simulink library "csu_tmp_tracker_messsage_processing_lib"  (R2014b)
settings: Solver=ode45  StartTime=0.0  StopTime=10.0  RelTol=1e-3
libraries: util_info_lib x1
settings Model: Creator=escrane  LastModifiedBy=mstewart

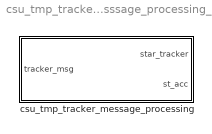
== system csu_tmp_tracker_messsage_processing_lib ==
  csu_tmp_tracker_message_processing : Subsystem

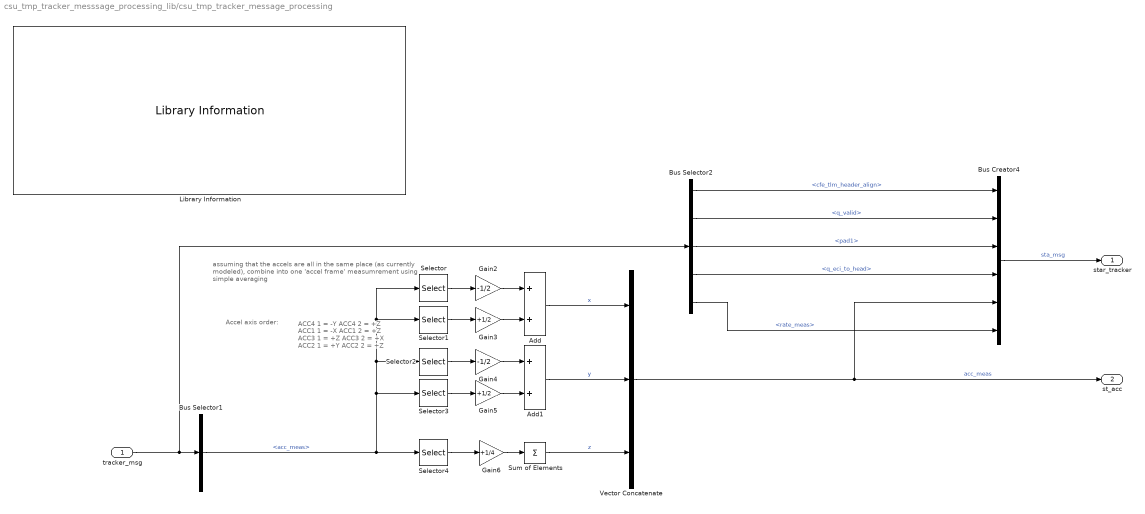
== system csu_tmp_tracker_messsage_processing_lib/csu_tmp_tracker_message_processing ==
  note: Accel axis order:
  note: assuming that the accels are all in the same place
      | (as currently modeled), combine into one 'accel frame'
      | measumrement using simple averaging
  note: ACC4 1 = -Y
      | ACC4 2 = +Z
      | ACC1 1 = -X
      | ACC1 2 = +Z
      | ACC3 1 = +Z
      | ACC3 2 = +X
      | ACC2 1 = +Y
      | ACC2 2 = +Z
  tracker_msg : Inport
  Add : Sum
  Add1 : Sum
  Bus Creator4 : BusCreator  Inputs=6
  Bus Selector1 : BusSelector  OutputSignals=acc_meas
  Bus Selector2 : BusSelector  OutputSignals=cfe_tlm_header_align,q_valid,pad1,q_eci_to_head,rate_meas
  Gain2 : Gain  Gain=-1/2
  Gain3 : Gain  Gain=+1/2
  Gain4 : Gain  Gain=-1/2
  Gain5 : Gain  Gain=+1/2
  Gain6 : Gain  Gain=+1/4
  Library Information : util_info_lib/Library Information  owner='escrane'
  Selector : Selector  NumberOfDimensions=2  InputPortWidth=3  IndexOptions=Select all,Index vector (dialog)  Indices=[3],[ 3 ]  OutputSizes=1,1
  Selector1 : Selector  NumberOfDimensions=2  InputPortWidth=3  IndexOptions=Select all,Index vector (dialog)  Indices=[6],[6]  OutputSizes=1,1
  Selector2 : Selector  NumberOfDimensions=2  InputPortWidth=3  IndexOptions=Select all,Index vector (dialog)  Indices=[1],[1]  OutputSizes=1,1
  Selector3 : Selector  NumberOfDimensions=2  InputPortWidth=3  IndexOptions=Select all,Index vector (dialog)  Indices=[7],[7]  OutputSizes=1,1
  Selector4 : Selector  NumberOfDimensions=2  InputPortWidth=3  IndexOptions=Select all,Index vector (dialog)  Indices=[2 4 5 8],[2 4 5 8]  OutputSizes=1,1
  Sum of Elements : Sum  Inputs=+  CollapseMode=Specified dimension  CollapseDim=2
  Vector Concatenate : Concatenate  NumInputs=3  Mode=Multidimensional array  ConcatenateDimension=2
  star_tracker : Outport
  st_acc : Outport  Port=2
  wires:
  Bus Creator4/1 -> star_tracker/1  "sta_msg"
  Bus Selector2/1 -> Bus Creator4/1  "<cfe_tlm_header_align>"
  Bus Selector2/2 -> Bus Creator4/2  "<q_valid>"
  Bus Selector2/3 -> Bus Creator4/3  "<pad1>"
  Bus Selector2/4 -> Bus Creator4/4  "<q_eci_to_head>"
  Bus Selector2/5 -> Bus Creator4/6  "<rate_meas>"
  tracker_msg/1 -> Bus Selector1/1, Bus Selector2/1
  Bus Selector1/1 -> Selector4/1, Selector2/1, Selector1/1, Selector/1, Selector3/1  "<acc_meas>"
  Selector/1 -> Gain2/1
  Selector1/1 -> Gain3/1
  Gain2/1 -> Add/1
  Gain3/1 -> Add/2
  Add/1 -> Vector Concatenate/1  "x"
  Selector2/1 -> Gain4/1
  Selector3/1 -> Gain5/1
  Gain4/1 -> Add1/1
  Gain5/1 -> Add1/2
  Add1/1 -> Vector Concatenate/2  "y"
  Selector4/1 -> Gain6/1
  Gain6/1 -> Sum of Elements/1
  Sum of Elements/1 -> Vector Concatenate/3  "z"
  Vector Concatenate/1 -> Bus Creator4/5, st_acc/1  "acc_meas"
